simulink model "ACC_Sample"  (R2024b)
settings: Solver=VariableStepAuto  StartTime=0.0  StopTime=nCount*T*Td  RelTol=1e-3
values from neighbouring files (symbols this model uses):
  T = 0.1    [File.mat]
  Td = 4    [File.mat]
  uRange = [-6474.6 6474.6]    [File.mat]
  xRange = [0  100; 10  30]    [File.mat]
  zRange = [16 31]    [File.mat]
libraries: autolibshared x1
settings Model: Creator=12775  LastModifiedBy=12775

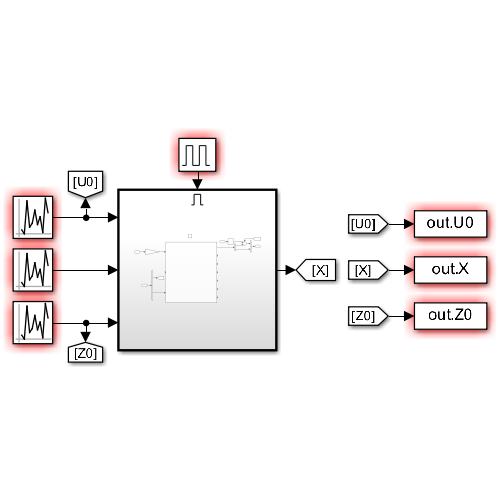
[thumbnail: Simulink's stored preview of the top-level diagram]
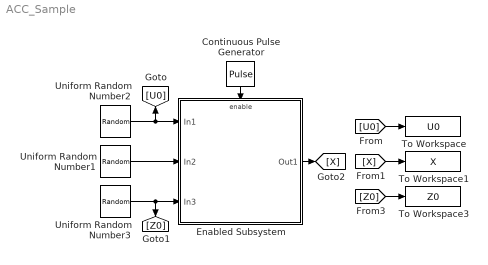
== system ACC_Sample ==
  Continuous Pulse Generator : DiscretePulseGenerator  PulseType=Time based  Period=T*Td  PulseWidth=75
  Enabled Subsystem : Subsystem  TreatAsAtomicUnit=on
  To Workspace : ToWorkspace  VariableName=U0  SampleTime=T
  To Workspace1 : ToWorkspace  VariableName=X  SampleTime=T
  To Workspace3 : ToWorkspace  VariableName=Z0  SampleTime=T
  Uniform Random Number1 : UniformRandomNumber  Minimum=xRange(:,1)  Maximum=xRange(:,2)  Seed=[1,2]  SampleTime=T*Td
  Uniform Random Number2 : UniformRandomNumber  Minimum=uRange(1)  Maximum=uRange(2)  SampleTime=T
  Uniform Random Number3 : UniformRandomNumber  Minimum=zRange(:,1)  Maximum=zRange(:,2)  Seed=3  SampleTime=T*Td
  wires:
  Enabled Subsystem/1(Out1) -> [X]
  [Z0] -> To Workspace3/1
  Continuous Pulse Generator/1 -> Enabled Subsystem/Enable
  Uniform Random Number3/1 -> Enabled Subsystem/3(In3), [Z0]
  [U0] -> To Workspace/1
  Uniform Random Number1/1 -> Enabled Subsystem/2(In2)
  Uniform Random Number2/1 -> Enabled Subsystem/1(In1), [U0]
  [X] -> To Workspace1/1

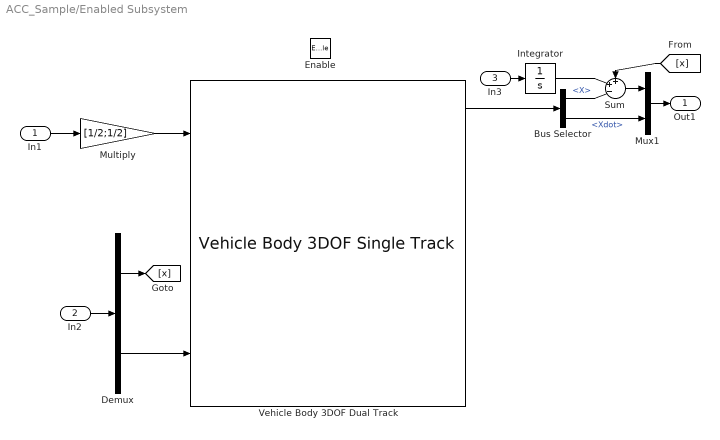
== system ACC_Sample/Enabled Subsystem ==
  In1 : Inport
  In2 : Inport  Port=2
  In3 : Inport  Port=3
  Enable : EnablePort  StatesWhenEnabling=reset
  Bus Selector : BusSelector  OutputSignals=InertFrm.Cg.Disp.X,InertFrm.Cg.Vel.Xdot
  Demux : Demux  Outputs=2
  Integrator : Integrator
  Multiply : Gain  Gain=[1/2;1/2]
  Mux1 : Mux  Inputs=2
  Sum : Sum  Inputs=++-|
  Vehicle Body 3DOF Dual Track : autolibshared/Vehicle Body 3DOF Single Track  trackMode=Dual  inputMode=External longitudinal forces  frontSteerMode=off  rearSteerMode=off  windMode=off  muMode=off  extFMode=off  extMMode=off  htchFMode=off  htchMMode=off  extXo=off  extpsio=off  extxdoto=on  extro=off  extYo=off  extTamb=off  extydoto=off  aMode=2  NF=2  NR=2  m=2000  a=1.4  b=1.6  h=0.35  dh=1  hh=0.2  X_o=0  xdot_o=0  CalphaMode=off  sigmaMode=off  d=0  hl=0  w=[1.4,1.4]  Cy_f=12e3  Cy_r=11e3  sigma_f=.1  sigma_r=.1  alpha_f_brk=[-.1 .1]  Cy_f_data=[-9e3 9e3]  alpha_r_brk=[-.1 .1]  Cy_r_data=[-9e3 9e3]  Y_o=0  ydot_o=0  Izz=4000  psi_o=0  r_o=0  Af=2  Cd=.3  Cl=.1  Cpm=.1  beta_w=[0 0.01:0.01:0.3]  Cs=[0:0.03:0.9]  Cym=[0 1e-6:0.01:0.3]  Pabs=101325  Tair=273  g=9.81  mu=1  xdot_tol=.01  Fznom=5000  Fxtire_sat=7e4  Fytire_sat=7e4  longOff=0  latOff=0  vertOff=0  wrapAng=off
      settings: LibrarySourceBlock=vehdynlibeom/Vehicle Body 3DOF Dual Track
  Out1 : Outport
  wires:
  In2/1 -> Demux/1
  Sum/1 -> Mux1/1
  Demux/1 -> [x]
  In3/1 -> Integrator/1
  Bus Selector/1 -> Sum/3  "<X>"
  [x] -> Sum/1
  Vehicle Body 3DOF Dual Track/1 -> Bus Selector/1
  Multiply/1 -> Vehicle Body 3DOF Dual Track/1
  Integrator/1 -> Sum/2
  Mux1/1 -> Out1/1
  Bus Selector/2 -> Mux1/2  "<Xdot>"
  Demux/2 -> Vehicle Body 3DOF Dual Track/3
  In1/1 -> Multiply/1
